simulink library "Weather_from_Workspace"  (R2018b)
settings: Solver=ode45  StartTime=0.0  StopTime=10.0  RelTol=1e-3  EnableMultiTasking=on
libraries: carnot x1
settings Model: Creator=lena.frank  LastModifiedBy=drhf
settings DataIOCC: LimitDataPoints=on  SaveFormat=Array  SignalLoggingSaveFormat=ModelDataLogs
settings OptimizationCC: ExpressionDepthLimit=2147483647  LifeSpan=inf
settings DebuggingCC: UnderspecifiedInitializationDetection=Classic  MergeDetectMultiDrivingBlocksExec=none  SolverPrmCheckMsg=warning  FcnCallInpInsideContextMsg=warning  StateNameClashWarn=warning  SFUnexpectedBacktrackingDiag=warning  SFNoUnconditionalDefaultTransitionDiag=warning  SFExecutionAtInitializationDiag=none
settings HardwareCC: ProdBitPerPointer=32  ProdBitPerSizeT=32  ProdBitPerPtrDiffT=32  ProdLargestAtomicFloat=None  ProdIntDivRoundTo=Undefined  ProdEndianess=Unspecified  ProdWordSize=32  ProdHWDeviceType=32-bit Generic
settings ModelReferenceCC: PropagateSignalLabelsOutOfModel=off
settings SFSimCC: SimUseLocalCustomCode=off
settings RTWCC: RTWUseLocalCustomCode=off
settings CodeAppCC: StateflowObjectComments=on
settings GRTTargetCC: TargetLangStandard=C89/C90 (ANSI)  GeneratePreprocessorConditionals=Disable all  CombineOutputUpdateFcns=off  GRTInterface=on
settings ConfigComp: CovMetricSettings=dw  CovHtmlReporting=on  CovSaveCumulativeToWorkspaceVar=on  CovSaveSingleToWorkspaceVar=on  CovExternalEMLEnable=off

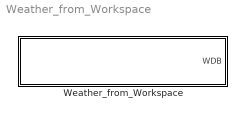
== system Weather_from_Workspace ==
  Weather_from_Workspace : Subsystem  mask(weather from workspace){file=DE_TRY2010_06_averageYear}
      mask prompts: file "Name of variable"
      mask help:
      | Input block for external weather data variables. The variable must be available in the workspace. A "From Workspace" Block is used in the subsystem.
      | A Unit-Delay with the timestep of the weather data forces the model to a maximum timestep equal to the data acquisiton timestep.
      | Remark: Be carefull when using the TRY Data 2010 for Germany. The files are public and can be found in the parameter_set folder of this block. But there are bugs is the solar radiation data.
      mask init:
      | % set variable name in the From Workspace block
      | set_param([gcb '/From_Workspace'], 'VariableName', file);
      | % sample time is timestep of weather data
      | t_sample = evalin('base',eval(['''',eval('file'),'(3,1)'''])) - evalin('base',eval(['''',eval('file'),'(2,1)''']));
      mask Help: web(fullfile(path_carnot('help'),'Weather_from_Workspace.html'),'-helpbrowser')
      mask Display: disp(file)

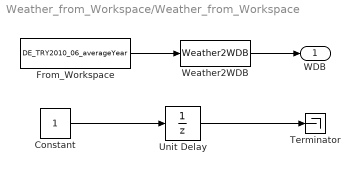
== system Weather_from_Workspace/Weather_from_Workspace ==
  Constant : Constant
  From_Workspace : FromWorkspace  VariableName=DE_TRY2010_06_averageYear  SampleTime=0  OutputAfterFinalValue=Setting to zero
  Terminator : Terminator
  Unit Delay : UnitDelay  SampleTime=t_sample
  Weather2WDB : carnot/Toolbox/Weather2WDB
      settings: SourceProductName=Carnot
  WDB : Outport
  wires:
  Weather2WDB/1 -> WDB/1
  Unit Delay/1 -> Terminator/1
  Constant/1 -> Unit Delay/1
  From_Workspace/1 -> Weather2WDB/1
